simulink model "VVI_Assignment1"  (R2020a)
settings: Solver=FixedStepAuto  StartTime=0.0  StopTime=10.0  FixedStep=1e-3  RelTol=1e-3  EnableMultiTasking=on
undefined symbols (not defined in the file): D1, D10, D11, D12, D13, D2, D3, D5, D8, D9, PTA0, PTA1, PTA2, PTB9, PTC17, PTC4, PTD0, PTD1, PTD2, PTD3
libraries: frdmk64flib x10
settings Model: ExtModeTrigDuration=5  Creator=wwwsh  LastModifiedBy=wwwsh
settings OptimizationCC: EnhancedBackFolding=on  PassReuseOutputArgsAs=Individual arguments  ZeroExternalMemoryAtStartup=off  ZeroInternalMemoryAtStartup=off  MaxStackSize=64  OptimizeBlockOrder=speed  DifferentSizesBufferReuse=on  OptimizationCustomize=off  EfficientTunableParamExpr=on
settings DebuggingCC: ParameterTunabilityLossMsg=error
settings HardwareCC: ProdBitPerPointer=32  ProdBitPerSizeT=32  ProdBitPerPtrDiffT=32  ProdLargestAtomicInteger=Long  ProdLargestAtomicFloat=Double  ProdWordSize=32  ProdHWDeviceType=ARM Compatible->ARM Cortex
settings SFSimCC: MATLABDynamicMemAlloc=off
settings RTWCC: SystemTargetFile=ert.tlc  HardwareBoard=NXP FRDM-K64F  TemplateMakefile=ert_default_tmf  Toolchain=GNU Tools for ARM Embedded Processors
settings CodeAppCC: ForceParamTrailComments=on  IgnoreCustomStorageClasses=off  OperatorAnnotations=on  SimulinkDataObjDesc=on  SFDataObjDesc=on  InsertBlockDesc=on

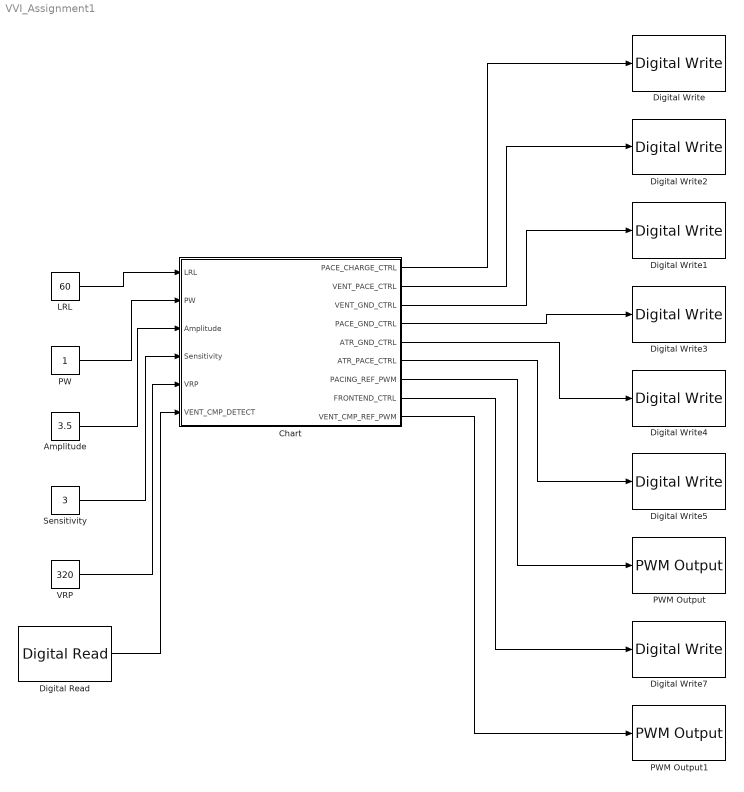
== system VVI_Assignment1 ==
  Amplitude : Constant  Value=3.5
  Chart : Stateflow chart  TreatAsAtomicUnit=on
  Digital Read : frdmk64flib/Digital Read  Whichpin=PTC17 (D1)  SampleTime=-1
  Digital Write : frdmk64flib/Digital Write  Whichpin=PTB9 (D2)
  Digital Write1 : frdmk64flib/Digital Write  Whichpin=PTD3 (D12)
  Digital Write2 : frdmk64flib/Digital Write  Whichpin=PTC4 (D9)
  Digital Write3 : frdmk64flib/Digital Write  Whichpin=PTD0 (D10)
  Digital Write4 : frdmk64flib/Digital Write  Whichpin=PTD2 (D11)
  Digital Write5 : frdmk64flib/Digital Write  Whichpin=PTA0 (D8)
  Digital Write7 : frdmk64flib/Digital Write  Whichpin=PTD1 (D13)
  LRL : Constant  Value=60
  PW : Constant
  PWM Output : frdmk64flib/PWM Output  Whichpin=PTA2 (D5)  InitialFrequency=2000  InitialDutyCycle=0
  PWM Output1 : frdmk64flib/PWM Output  Whichpin=PTA1 (D3)  InitialFrequency=2000  InitialDutyCycle=0
  Sensitivity : Constant  Value=3
  VRP : Constant  Value=320
  wires:
  LRL/1 -> Chart/1(LRL)
  PW/1 -> Chart/2(PW)
  Amplitude/1 -> Chart/3(Amplitude)
  Sensitivity/1 -> Chart/4(Sensitivity)
  VRP/1 -> Chart/5(VRP)
  Digital Read/1 -> Chart/6(VENT_CMP_DETECT)
  Chart/1(PACE_CHARGE_CTRL) -> Digital Write/1
  Chart/2(VENT_PACE_CTRL) -> Digital Write2/1
  Chart/3(VENT_GND_CTRL) -> Digital Write1/1
  Chart/4(PACE_GND_CTRL) -> Digital Write3/1
  Chart/5(ATR_GND_CTRL) -> Digital Write4/1
  Chart/6(ATR_PACE_CTRL) -> Digital Write5/1
  Chart/7(PACING_REF_PWM) -> PWM Output/1
  Chart/8(FRONTEND_CTRL) -> Digital Write7/1
  Chart/9(VENT_CMP_REF_PWM) -> PWM Output1/1

== stateflow chart VVI_Assignment1/Chart ==
  state VVI_Charge
    entry:
    % Charges primary capacitor
    ATR_PACE_CTRL = false;
    VENT_PACE_CTRL = false;
    PACING_REF_PWM = Amplitude * 20;
    PACE_CHARGE_CTRL = true;
    FRONTEND_CTRL = false;
    % Discharging blocking capacitor
    PACE_GND_CTRL = true;
    VENT_PACE_CTRL = false;
    ATR_PACE_CTRL = false;
    ATR_GND_CTRL = false;
    VENT_GND_CTRL = true;
  state VVI_Pace
    entry:
    % Paces ventricle
    PACE_CHARGE_CTRL = false;
    PACE_GND_CTRL = true;
    ATR_PACE_CTRL = false;
    ATR_GND_CTRL = false;
    VENT_GND_CTRL = false;
    VENT_PACE_CTRL = true;
    FRONTEND_CTRL = true;
    PACING_REF_PWM = Amplitude * 20;
  state VVI_Sense
    entry:
    PACE_CHARGE_CTRL = true;
    PACE_GND_CTRL = true;
    VENT_GND_CTRL = true;
    VENT_PACE_CTRL = false;
    FRONTEND_CTRL = true;
    PACING_REF_PWM = Amplitude * 20;
    VENT_CMP_REF_PWM = (Sensitivity)*20;
  (default) -> VVI_Charge
  VVI_Charge -> VVI_Pace [order 2] : after((60000/LRL) - VRP - PW, msec)
  VVI_Pace -> VVI_Sense : after(PW, msec)
  VVI_Sense -> VVI_Charge : after(VRP, msec)
  VVI_Charge -> VVI_Sense [order 1] : [VENT_CMP_DETECT == true]{(60000/LRL) - VRP}
  data: LRL input; PW input; Amplitude input; Sensitivity input; VRP input; VENT_CMP_DETECT input; PACE_CHARGE_CTRL output; VENT_PACE_CTRL output; VENT_GND_CTRL output; PACE_GND_CTRL output; ATR_GND_CTRL output; ATR_PACE_CTRL output; PACING_REF_PWM output; FRONTEND_CTRL output; VENT_CMP_REF_PWM output
